simulink model "sub1"  (R2021b)
settings: Solver=FixedStepDiscrete  StartTime=0.0  StopTime=10.0  RelTol=1e-3
libraries: SimulinkLibrary x3
settings Model: Creator=AnusreeSaji  LastModifiedBy=AnusreeSaji

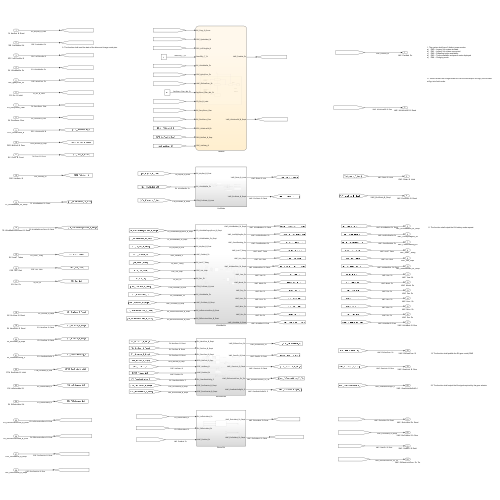
[thumbnail: Simulink's stored preview of the top-level diagram]
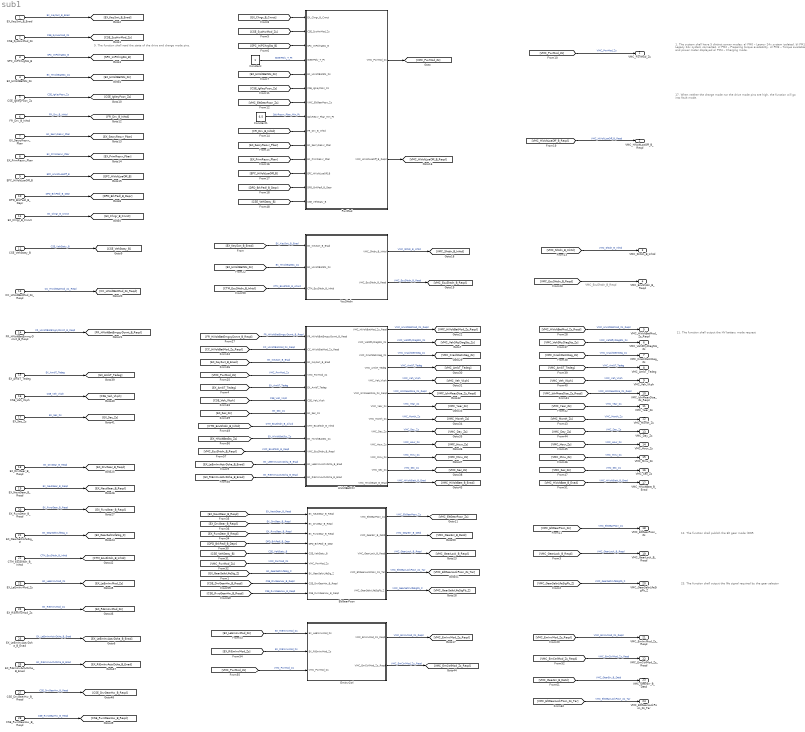
== system sub1 ==
  note: VMC_EcuShtdn_B_Reqd
  note: 11. The function shall output the HV battery mode request
  note: 9. The function shall read the state of the drive and charge mode pins.
  note: 17. When neither the charge mode nor the drive mode pins are high, the function will go into fault mode.
  note: 12. The function shall publish the Elt gear mode (DNR
  note: 1. The system shall have 5 distinct power modes:
      | a)	PM0 – Legacy 24v system isolated.
      | b)	PM1 – Legacy 24v system connected.
      | c)	PM2 – Preparing torque availability.
      | d)	PM3 – Torque available and power meter displayed
      | e)	PM4 – Charging mode.
  note: 23. The function shall output the life signal required by the gear selector
  EX_KeySwt_B_Enad : Inport
  CSE_SysHwMod_Zs : Inport  Port=2
  SPC_IniPChrgSts_B : Inport  Port=3
  EX_HiVoltBatSts_Zs : Inport  Port=4
  CSE_IgKeyPosn_Zs : Inport  Port=5
  FR_Drv_B_Inhtd : Inport  Port=6
  EX_SecryResvr_Pbar : Inport  Port=7
  EX_PrimResvr_Pbar : Inport  Port=8
  EPC_HiVoltLoaOff_B : Inport  Port=9
  DPD_BrkPedl_B_Depr : Inport  Port=10
  EX_Chrgr_B_Cnnct : Inport  Port=11
  CSE_VehStaty_B : Inport  Port=12
  CC_HiVoltBatMod_Zs_Reqd : Inport  Port=13
  FR_HiVoltBatEmgcyDcnnt_B_Reqd : Inport  Port=14
  EX_AmbT_Tedeg : Inport  Port=15
  CSE_Veh_Vkph : Inport  Port=16
  EX_Sec_Zs : Inport  Port=17
  EX_DrvGear_B_Reqd : Inport  Port=18
  EX_NeutGear_B_Reqd : Inport  Port=19
  EX_RvrsGear_B_Reqd : Inport  Port=20
  EX_GearSeltrLifeSig_Z : Inport  Port=21
  CTM_EcuShtdn_B_Inhtd : Inport  Port=22
  EX_LeEmInvMod_Zs : Inport  Port=23
  EX_RiEmInvMod_Zs : Inport  Port=24
  EX_LeEmInvActvDcha_B_Enad : Inport  Port=25
  EX_RiEmInvActvDcha_B_Enad : Inport  Port=26
  CSE_DrvGearHw_B_Reqd : Inport  Port=27
  CSE_RvrsGearHw_B_Reqd : Inport  Port=28
  Constant : Constant
  Constant1 : Constant  Value=6.5
  EltGearPosn : Subsystem
  EmInvCtrl : Subsystem
  HiVoltBatCtrl : Subsystem
  PwrMod : Stateflow chart  TreatAsAtomicUnit=on
  VcuShtdn : Subsystem
  VMC_PwrMod_Zs : Outport  OutDataTypeStr=single
  VMC_HiVoltLoaOff_B_Reqd : Outport  Port=2
  VMC_Shtdn_B_Inhtd : Outport  Port=3
  VMC_EcuShtdn_B_Reqd : Outport  Port=4
  VMC_HiVoltBatMod_Zs_Reqd : Outport  Port=5
  VMC_VehSftyDiagSts_Zs : Outport  Port=6
  VMC_CrashDetnNeg_Zs : Outport  Port=7
  VMC_AmbT_Tedeg : Outport  Port=8
  VMC_Veh_Vkph : Outport  Port=9
  VMC_IslnMeasDisa_Zs_Reqd : Outport  Port=10
  VMC_Year_Zs : Outport  Port=11
  VMC_Month_Zs : Outport  Port=12
  VMC_Day_Zs : Outport  Port=13
  VMC_Hour_Zs : Outport  Port=14
  VMC_Minu_Zs : Outport  Port=15
  VMC_Sec_Zs : Outport  Port=16
  VMC_HiVoltBatt_B_Enad : Outport  Port=17
  VMC_EltGearPosn_Zs : Outport  Port=18
  VMC_GearLock_B_Reqd : Outport  Port=19
  VMC_GearSeltrLifeSigFb_Z : Outport  Port=20
  VMC_EmInvMod_Zs_Reqd : Outport  Port=21
  VMC_EmCtrlMod_Zs_Reqd : Outport  Port=22
  VMC_GearErr_B_Detd : Outport  Port=23
  VMC_EltGearLockPosn_Zs_Tar : Outport  Port=24
  wires:
  CSE_IgKeyPosn_Zs/1 -> [CSE_IgKeyPosn_Zs]  "CSE_IgKeyPosn_Zs"
  SPC_IniPChrgSts_B/1 -> [SPC_IniPChrgSts_B]  "SPC_IniPChrgSts_B"
  [CSE_SysHwMod_Zs] -> PwrMod/2(CSE_SysHwMod_Zs)
  EX_HiVoltBatSts_Zs/1 -> [EX_HiVoltBatSts_Zs]  "EX_HiVoltBatSts_Zs"
  [VMC_PwrMod_Zs] -> EltGearPosn/6(VMC_PwrMod_Zs)  "VMC_PwrMod_Zs"
  [VMC_EltGearPosn_Zs] -> PwrMod/7(VMC_EltGearPosn_Zs)
  CSE_SysHwMod_Zs/1 -> [CSE_SysHwMod_Zs]  "CSE_SysHwMod_Zs"
  PwrMod/1(VMC_PwrMod_Zs) -> [VMC_PwrMod_Zs]
  EX_RvrsGear_B_Reqd/1 -> [EX_RvrsGear_B_Reqd]  "EX_RvrsGear_B_Reqd"
  CSE_RvrsGearHw_B_Reqd/1 -> [CSE_RvrsGearHw_B_Reqd]  "CSE_RvrsGearHw_B_Reqd"
  [CSE_VehStaty_B] -> EltGearPosn/5(CSE_VehStaty_B)  "CSE_VehStaty_B"
  [SPC_IniPChrgSts_B] -> PwrMod/3(SPC_IniPChrgSts_B)
  Constant/1 -> PwrMod/4(SteerPDly_T_Pt)  "SteerPDly_T_Pt"
  [EX_HiVoltBatSts_Zs] -> VcuShtdn/2(EX_HiVoltBatSts_Zs)  "EX_HiVoltBatSts_Zs"
  Constant1/1 -> PwrMod/8(SplyResvr_Pbar_Min_Pt)  "SplyResvr_Pbar_Min_Pt"
  [EX_Chrgr_B_Cnnct] -> PwrMod/1(EX_Chrgr_B_Cnnct)
  HiVoltBatCtrl/12(VMC_Sec_Zs) -> [VMC_Sec_Zs]  "VMC_Sec_Zs"
  VcuShtdn/1(VMC_Shtdn_B_Inhtd) -> [VMC_Shtdn_B_Inhtd]  "VMC_Shtdn_B_Inhtd"
  [CSE_IgKeyPosn_Zs] -> PwrMod/6(CSE_IgKeyPosn_Zs)
  EltGearPosn/5(VMC_GearSeltrLifeSigFb_Z) -> [VMC_GearSeltrLifeSigFb_Z]  "VMC_GearSeltrLifeSigFb_Z"
  CC_HiVoltBatMod_Zs_Reqd/1 -> [CC_HiVoltBatMod_Zs_Reqd]  "CC_HiVoltBatMod_Zs_Reqd"
  [EX_SecryResvr_Pbar] -> PwrMod/10(EX_SecryResvr_Pbar)
  [CSE_Veh_Vkph] -> HiVoltBatCtrl/6(CSE_Veh_Vkph)  "CSE_Veh_Vkph"
  [VMC_PwrMod_Zs] -> EmInvCtrl/3(VMC_PwrMod_Zs)  "VMC_PwrMod_Zs"
  [VMC_PwrMod_Zs] -> VMC_PwrMod_Zs/1  "VMC_PwrMod_Zs"
  [EX_HiVoltBatSts_Zs] -> PwrMod/5(EX_HiVoltBatSts_Zs)
  [DPD_BrkPedl_B_Depr] -> PwrMod/13(DPD_BrkPedl_B_Depr)
  [EX_HiVoltBatSts_Zs] -> HiVoltBatCtrl/9(EX_HiVoltBatSts_Zs)  "EX_HiVoltBatSts_Zs"
  [VMC_Sec_Zs] -> VMC_Sec_Zs/1  "VMC_Sec_Zs"
  EltGearPosn/3(VMC_GearLock_B_Reqd) -> [VMC_GearLock_B_Reqd]  "VMC_GearLock_B_Reqd"
  DPD_BrkPedl_B_Depr/1 -> [DPD_BrkPedl_B_Depr]  "DPD_BrkPedl_B_Depr"
  CSE_VehStaty_B/1 -> [CSE_VehStaty_B]  "CSE_VehStaty_B"
  FR_Drv_B_Inhtd/1 -> [FR_Drv_B_Inhtd]  "FR_Drv_B_Inhtd"
  EX_RiEmInvActvDcha_B_Enad/1 -> [EX_RiEmInvActvDcha_B_Enad]  "EX_RiEmInvActvDcha_B_Enad"
  [VMC_GearLock_B_Reqd] -> VMC_GearLock_B_Reqd/1  "VMC_GearLock_B_Reqd"
  [VMC_EmInvMod_Zs_Reqd] -> VMC_EmInvMod_Zs_Reqd/1  "VMC_EmInvMod_Zs_Reqd"
  [VMC_EltGearLockPosn_Zs_Tar] -> VMC_EltGearLockPosn_Zs_Tar/1  "VMC_EltGearLockPosn_Zs_Tar"
  [VMC_HiVoltLoaOff_B_Reqd] -> VMC_HiVoltLoaOff_B_Reqd/1  "VMC_HiVoltLoaOff_B_Reqd"
  [EX_AmbT_Tedeg] -> HiVoltBatCtrl/5(EX_AmbT_Tedeg)  "EX_AmbT_Tedeg"
  EmInvCtrl/1(VMC_EmInvMod_Zs_Reqd) -> [VMC_EmInvMod_Zs_Reqd]  "VMC_EmInvMod_Zs_Reqd"
  EX_AmbT_Tedeg/1 -> [EX_AmbT_Tedeg]  "EX_AmbT_Tedeg"
  CSE_Veh_Vkph/1 -> [CSE_Veh_Vkph]  "CSE_Veh_Vkph"
  HiVoltBatCtrl/13(VMC_HiVoltBatt_B_Enad) -> [VMC_HiVoltBatt_B_Enad]  "VMC_HiVoltBatt_B_Enad"
  EPC_HiVoltLoaOff_B/1 -> [EPC_HiVoltLoaOff_B]  "EPC_HiVoltLoaOff_B"
  EX_RiEmInvMod_Zs/1 -> [EX_RiEmInvMod_Zs]  "EX_RiEmInvMod_Zs"
  [VMC_EmCtrlMod_Zs_Reqd] -> VMC_EmCtrlMod_Zs_Reqd/1  "VMC_EmCtrlMod_Zs_Reqd"
  CTM_EcuShtdn_B_Inhtd/1 -> [CTM_EcuShtdn_B_Inhtd]  "CTM_EcuShtdn_B_Inhtd"
  [CTM_EcuShtdn_B_Inhtd] -> VcuShtdn/3(CTM_EcuShtdn_B_Inhtd)  "CTM_EcuShtdn_B_Allwd"
  HiVoltBatCtrl/6(VMC_IslnMeasDisa_Zs_Reqd) -> [VMC_IslnMeasDisa_Zs_Reqd]  "VMC_IslnMeasDisa_Zs_Reqd"
  EX_LeEmInvActvDcha_B_Enad/1 -> [EX_LeEmInvActvDcha_B_Enad]  "EX_LeEmInvActvDcha_B_Enad"
  [EX_RiEmInvMod_Zs] -> EmInvCtrl/2(EX_RiEmInvMod_Zs)  "EX_RiEmInvMod_Zs"
  [EX_LeEmInvActvDcha_B_Enad] -> HiVoltBatCtrl/11(EX_LeEmInvActvDcha_B_Enad)  "EX_LeEmInvActvDcha_B_Enad"
  HiVoltBatCtrl/1(VMC_HiVoltBatMod_Zs_Reqd) -> [VMC_HiVoltBatMod_Zs_Reqd]  "VMC_HiVoltBatMod_Zs_Reqd"
  [VMC_CrashDetnNeg_Zs] -> VMC_CrashDetnNeg_Zs/1  "VMC_CrashDetnNeg_Zs"
  [FR_HiVoltBatEmgcyDcnnt_B_Reqd] -> HiVoltBatCtrl/1(FR_HiVoltBatEmgcyDcnnt_B_Reqd)  "FR_HiVoltBatEmgcyDcnnt_B_Reqd"
  [VMC_PwrMod_Zs] -> HiVoltBatCtrl/4(VMC_PwrMod_Zs)  "VMC_PwrMod_Zs"
  [VMC_HiVoltBatMod_Zs_Reqd] -> VMC_HiVoltBatMod_Zs_Reqd/1  "VMC_HiVoltBatMod_Zs_Reqd"
  [EX_LeEmInvMod_Zs] -> EmInvCtrl/1(EX_LeEmInvMod_Zs)  "EX_RiEmInvMod_Zs"
  [VMC_Minu_Zs] -> VMC_Minu_Zs/1  "VMC_Minu_Zs"
  EX_Chrgr_B_Cnnct/1 -> [EX_Chrgr_B_Cnnct]  "EX_Chrgr_B_Cnnct"
  [EX_DrvGear_B_Reqd] -> EltGearPosn/2(EX_DrvGear_B_Reqd)  "EX_DrvGear_B_Reqd"
  [CSE_DrvGearHw_B_Reqd] -> EltGearPosn/8(CSE_DrvGearHw_B_Reqd)  "CSE_DrvGearHw_B_Reqd"
  [EX_RvrsGear_B_Reqd] -> EltGearPosn/3(EX_RvrsGear_B_Reqd)  "EX_RvrsGear_B_Reqd"
  EltGearPosn/1(VMC_EltGearPosn_Zs) -> [VMC_EltGearPosn_Zs]  "VMC_EltGearPosn_Zs"
  FR_HiVoltBatEmgcyDcnnt_B_Reqd/1 -> [FR_HiVoltBatEmgcyDcnnt_B_Reqd]  "FR_HiVoltBatEmgcyDcnnt_B_Reqd"
  CSE_DrvGearHw_B_Reqd/1 -> [CSE_DrvGearHw_B_Reqd]  "CSE_DrvGearHw_B_Reqd"
  [EX_Sec_Zs] -> HiVoltBatCtrl/7(EX_Sec_Zs)  "EX_Sec_Zs"
  HiVoltBatCtrl/5(VMC_Veh_Vkph) -> [VMC_Veh_Vkph]  "VMC_Veh_Vkph"
  EX_KeySwt_B_Enad/1 -> [EX_KeySwt_B_Enad]  "EX_KeySwt_B_Enad"
  HiVoltBatCtrl/2(VMC_VehSftyDiagSts_Zs) -> [VMC_VehSftyDiagSts_Zs]  "VMC_VehSftyDiagSts_Zs"
  EX_LeEmInvMod_Zs/1 -> [EX_LeEmInvMod_Zs]  "EX_LeEmInvMod_Zs"
  [EX_KeySwt_B_Enad] -> HiVoltBatCtrl/3(EX_KeySwt_B_Enad)  "EX_KeySwt_B_Enad"
  HiVoltBatCtrl/3(VMC_CrashDetnNeg_Zs) -> [VMC_CrashDetnNeg_Zs]  "VMC_CrashDetnNeg_Zs"
  HiVoltBatCtrl/4(VMC_AmbT_Tedeg) -> [VMC_AmbT_Tedeg]  "VMC_AmbT_Tedeg"
  EltGearPosn/4(VMC_EltGearLockPosn_Zs_Tar) -> [VMC_EltGearLockPosn_Zs_Tar]  "VMC_EltGearLockPosn_Zs_Tar"
  [VMC_GearErr_B_Detd] -> VMC_GearErr_B_Detd/1  "VMC_GearErr_B_Detd"
  EltGearPosn/2(VMC_GearErr_B_Detd) -> [VMC_GearErr_B_Detd]  "VMC_GearErr_B_Detd"
  [VMC_Veh_Vkph] -> VMC_Veh_Vkph/1  "VMC_Veh_Vkph"
  HiVoltBatCtrl/7(VMC_Year_Zs) -> [VMC_Year_Zs]  "VMC_Year_Zs"
  EX_NeutGear_B_Reqd/1 -> [EX_NeutGear_B_Reqd]  "EX_NeutGear_B_Reqd"
  HiVoltBatCtrl/11(VMC_Minu_Zs) -> [VMC_Minu_Zs]  "VMC_Minu_Zs"
  [VMC_Month_Zs] -> VMC_Month_Zs/1  "VMC_Month_Zs"
  [VMC_AmbT_Tedeg] -> VMC_AmbT_Tedeg/1  "VMC_AmbT_Tedeg"
  EmInvCtrl/2(VMC_EmCtrlMod_Zs_Reqd) -> [VMC_EmCtrlMod_Zs_Reqd]  "VMC_EmCtrlMod_Zs_Reqd"
  [VMC_Day_Zs] -> VMC_Day_Zs/1  "VMC_Day_Zs"
  [CC_HiVoltBatMod_Zs_Reqd] -> HiVoltBatCtrl/2(CC_HiVoltBatMod_Zs_Reqd)  "CC_HiVoltBatMod_Zs_Reqd"
  [VMC_Hour_Zs] -> VMC_Hour_Zs/1  "VMC_Hour_Zs"
  [VMC_Year_Zs] -> VMC_Year_Zs/1  "VMC_Year_Zs"
  [DPD_BrkPedl_B_Depr] -> EltGearPosn/4(DPD_BrkPedl_B_Depr)  "DPD_BrkPedl_B_Depr"
  [VMC_Shtdn_B_Inhtd] -> VMC_Shtdn_B_Inhtd/1  "VMC_Shtdn_B_Inhtd"
  [VMC_HiVoltBatt_B_Enad] -> VMC_HiVoltBatt_B_Enad/1  "VMC_HiVoltBatt_B_Enad"
  [EX_NeutGear_B_Reqd] -> EltGearPosn/1(EX_NeutGear_B_Reqd)  "EX_NeutGear_B_Reqd"
  HiVoltBatCtrl/9(VMC_Day_Zs) -> [VMC_Day_Zs]  "VMC_Day_Zs"
  [CTM_EcuShtdn_B_Inhtd] -> HiVoltBatCtrl/8(CTM_EcuShtdn_B_Inhtd)  "CTM_EcuShtdn_B_Allwd"
  EX_GearSeltrLifeSig_Z/1 -> [EX_GearSeltrLifeSig_Z]  "EX_GearSeltrLifeSig_Z"
  [VMC_EltGearPosn_Zs] -> VMC_EltGearPosn_Zs/1  "VMC_EltGearPosn_Zs"
  HiVoltBatCtrl/8(VMC_Month_Zs) -> [VMC_Month_Zs]  "VMC_Month_Zs"
  EX_DrvGear_B_Reqd/1 -> [EX_DrvGear_B_Reqd]  "EX_DrvGear_B_Reqd"
  PwrMod/2(VMC_HiVoltLoaOff_B_Reqd) -> [VMC_HiVoltLoaOff_B_Reqd]
  VcuShtdn/2(VMC_EcuShtdn_B_Reqd) -> [VMC_EcuShtdn_B_Reqd]  "VMC_EcuShtdn_B_Reqd"
  [CSE_VehStaty_B] -> PwrMod/14(CSE_VehStaty_B)
  [FR_Drv_B_Inhtd] -> PwrMod/9(FR_Drv_B_Inhtd)
  [VMC_IslnMeasDisa_Zs_Reqd] -> VMC_IslnMeasDisa_Zs_Reqd/1  "VMC_IslnMeasDisa_Zs_Reqd"
  [EX_PrimResvr_Pbar] -> PwrMod/11(EX_PrimResvr_Pbar)
  EX_PrimResvr_Pbar/1 -> [EX_PrimResvr_Pbar]  "EX_PrimResvr_Pbar"
  EX_SecryResvr_Pbar/1 -> [EX_SecryResvr_Pbar]  "EX_SecryResvr_Pbar"
  [EX_RiEmInvActvDcha_B_Enad] -> HiVoltBatCtrl/12(EX_RiEmInvActvDcha_B_Enad)  "EX_RiEmInvActvDcha_B_Enad"
  EX_Sec_Zs/1 -> [EX_Sec_Zs]  "EX_Sec_Zs"
  [CSE_RvrsGearHw_B_Reqd] -> EltGearPosn/9(CSE_RvrsGearHw_B_Reqd)  "CSE_RvrsGearHw_B_Reqd"
  [EX_KeySwt_B_Enad] -> VcuShtdn/1(EX_KeySwt_B_Enad)  "EX_KeySwt_B_Enad"
  [EX_GearSeltrLifeSig_Z] -> EltGearPosn/7(EX_GearSeltrLifeSig_Z)  "EX_GearSeltrLifeSig_Z"
  [VMC_EcuShtdn_B_Reqd] -> VMC_EcuShtdn_B_Reqd/1
  HiVoltBatCtrl/10(VMC_Hour_Zs) -> [VMC_Hour_Zs]  "VMC_Hour_Zs"
  [EPC_HiVoltLoaOff_B] -> PwrMod/12(EPC_HiVoltLoaOff_B)
  [VMC_EcuShtdn_B_Reqd] -> HiVoltBatCtrl/10(VMC_EcuShtdn_B_Reqd)  "VMC_EcuShtdn_B_Reqd"
  [VMC_VehSftyDiagSts_Zs] -> VMC_VehSftyDiagSts_Zs/1  "VMC_VehSftyDiagSts_Zs"
  [VMC_GearSeltrLifeSigFb_Z] -> VMC_GearSeltrLifeSigFb_Z/1  "VMC_GearSeltrLifeSigFb_Z"

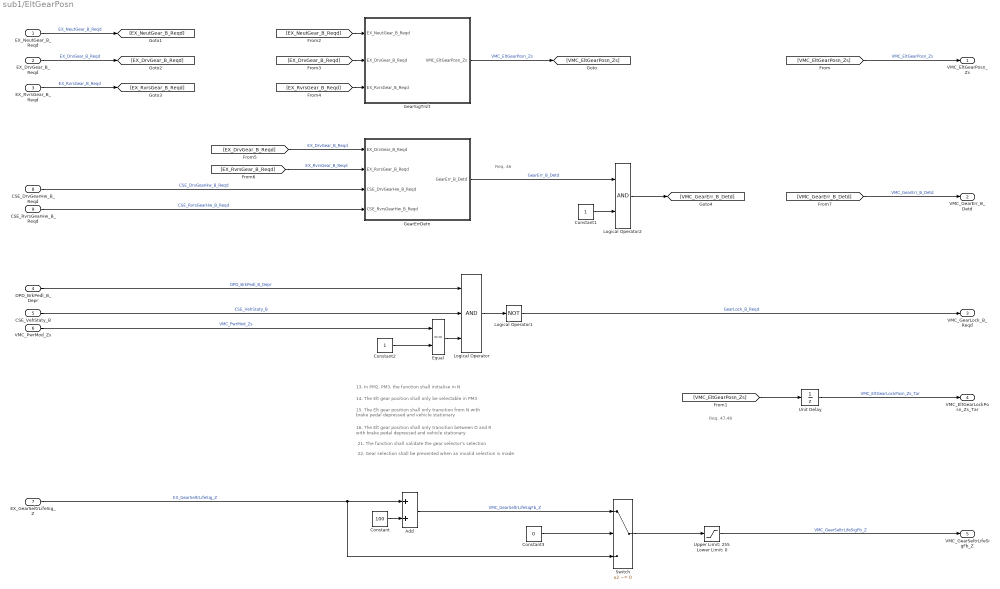
== system sub1/EltGearPosn ==
  note: 13. In PM2, PM3, the function shall initialise in N
  note: 14. The Elt gear position shall only be selectable in PM3
  note: 15. The Elt gear position shall only transition from N with brake pedal depressed and vehicle stationary
  note: 16. The Elt gear position shall only transition between D and R with brake pedal depressed and vehicle stationary
  note: 21. The function shall validate the gear selector’s selection
  note: 22. Gear selection shall be prevented when an invalid selection is made
  note: Req. 46
  note: Req. 47,48
  EX_NeutGear_B_Reqd : Inport
  EX_DrvGear_B_Reqd : Inport  Port=2
  EX_RvrsGear_B_Reqd : Inport  Port=3
  DPD_BrkPedl_B_Depr : Inport  Port=4
  CSE_VehStaty_B : Inport  Port=5
  VMC_PwrMod_Zs : Inport  Port=6
  EX_GearSeltrLifeSig_Z : Inport  Port=7
  CSE_DrvGearHw_B_Reqd : Inport  Port=8
  CSE_RvrsGearHw_B_Reqd : Inport  Port=9
  Add : Sum
  Constant : Constant  Value=100
  Constant1 : Constant
  Constant2 : Constant
  Constant3 : Constant  Value=0
  Equal : RelationalOperator  Operator===  OutDataTypeStr=boolean  RndMeth=Simplest
  GearErrDetn : Subsystem
  GearSigTrslt : Subsystem
  Logical Operator : Logic  Inputs=3  AllPortsSameDT=off  OutDataTypeStr=boolean
  Logical Operator1 : Logic  Operator=NOT  AllPortsSameDT=off  OutDataTypeStr=boolean
  Logical Operator2 : Logic  AllPortsSameDT=off  OutDataTypeStr=boolean
  Switch : Switch  Criteria=u2 ~= 0
  Unit Delay : UnitDelay  SampleTime=-1  HasFrameUpgradeWarning=on
  Upper Limit: 255 Lower Limit: 0 : Saturate  UpperLimit=100  LowerLimit=0
  VMC_EltGearPosn_Zs : Outport
  VMC_GearErr_B_Detd : Outport  Port=2
  VMC_GearLock_B_Reqd : Outport  Port=3
  VMC_EltGearLockPosn_Zs_Tar : Outport  Port=4
  VMC_GearSeltrLifeSigFb_Z : Outport  Port=5
  wires:
  Constant3/1 -> Switch/2
  Switch/1 -> Upper Limit: 255 Lower Limit: 0/1
  Add/1 -> Switch/1  "VMC_GearSeltrLifeSigFb_Z"
  Logical Operator2/1 -> [VMC_GearErr_B_Detd]
  [VMC_GearErr_B_Detd] -> VMC_GearErr_B_Detd/1  "VMC_GearErr_B_Detd"
  Constant1/1 -> Logical Operator2/2
  GearErrDetn/1(GearErr_B_Detd) -> Logical Operator2/1  "GearErr_B_Detd"
  CSE_DrvGearHw_B_Reqd/1 -> GearErrDetn/3(CSE_DrvGearHw_B_Reqd)  "CSE_DrvGearHw_B_Reqd"
  CSE_RvrsGearHw_B_Reqd/1 -> GearErrDetn/4(CSE_RvrsGearHw_B_Reqd)  "CSE_RvrsGearHw_B_Reqd"
  [EX_RvrsGear_B_Reqd] -> GearErrDetn/2(EX_RvrsGear_B_Reqd)  "EX_RvrsGear_B_Reqd"
  [EX_DrvGear_B_Reqd] -> GearErrDetn/1(EX_DrvGear_B_Reqd)  "EX_DrvGear_B_Reqd"
  [EX_RvrsGear_B_Reqd] -> GearSigTrslt/3(EX_RvrsGear_B_Reqd)
  [EX_DrvGear_B_Reqd] -> GearSigTrslt/2(EX_DrvGear_B_Reqd)
  [EX_NeutGear_B_Reqd] -> GearSigTrslt/1(EX_NeutGear_B_Reqd)
  Unit Delay/1 -> VMC_EltGearLockPosn_Zs_Tar/1  "VMC_EltGearLockPosn_Zs_Tar"
  [VMC_EltGearPosn_Zs] -> Unit Delay/1
  [VMC_EltGearPosn_Zs] -> VMC_EltGearPosn_Zs/1  "VMC_EltGearPosn_Zs"
  Upper Limit: 255 Lower Limit: 0/1 -> VMC_GearSeltrLifeSigFb_Z/1  "VMC_GearSeltrLifeSigFb_Z"
  Constant/1 -> Add/2
  EX_GearSeltrLifeSig_Z/1 -> Add/1, Switch/3  "EX_GearSeltrLifeSig_Z"
  EX_RvrsGear_B_Reqd/1 -> [EX_RvrsGear_B_Reqd]  "EX_RvrsGear_B_Reqd"
  EX_DrvGear_B_Reqd/1 -> [EX_DrvGear_B_Reqd]  "EX_DrvGear_B_Reqd"
  Logical Operator1/1 -> VMC_GearLock_B_Reqd/1  "GearLock_B_Reqd"
  VMC_PwrMod_Zs/1 -> Equal/1  "VMC_PwrMod_Zs"
  Logical Operator/1 -> Logical Operator1/1
  CSE_VehStaty_B/1 -> Logical Operator/2  "CSE_VehStaty_B"
  GearSigTrslt/1(VMC_EltGearPosn_Zs) -> [VMC_EltGearPosn_Zs]  "VMC_EltGearPosn_Zs"
  Equal/1 -> Logical Operator/3
  Constant2/1 -> Equal/2
  EX_NeutGear_B_Reqd/1 -> [EX_NeutGear_B_Reqd]  "EX_NeutGear_B_Reqd"
  DPD_BrkPedl_B_Depr/1 -> Logical Operator/1  "DPD_BrkPedl_B_Depr"

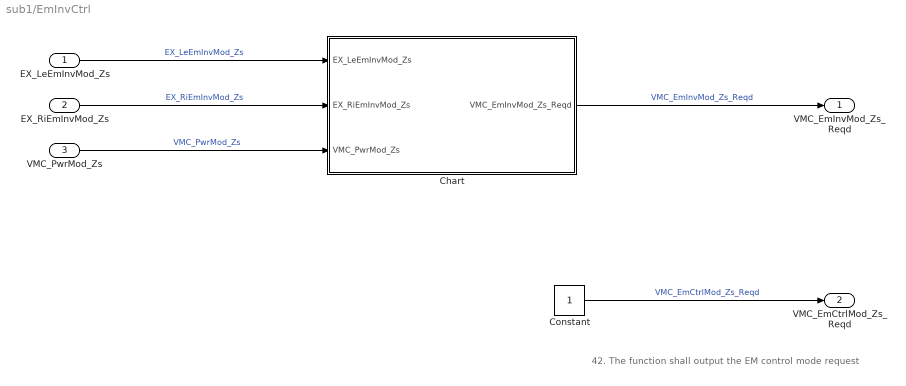
== system sub1/EmInvCtrl ==
  note: 42. The function shall output the EM control mode request
  EX_LeEmInvMod_Zs : Inport
  EX_RiEmInvMod_Zs : Inport  Port=2
  VMC_PwrMod_Zs : Inport  Port=3
  Chart : Stateflow chart  TreatAsAtomicUnit=on
  Constant : Constant
  VMC_EmInvMod_Zs_Reqd : Outport
  VMC_EmCtrlMod_Zs_Reqd : Outport  Port=2
  wires:
  Constant/1 -> VMC_EmCtrlMod_Zs_Reqd/1  "VMC_EmCtrlMod_Zs_Reqd"
  VMC_PwrMod_Zs/1 -> Chart/3(VMC_PwrMod_Zs)  "VMC_PwrMod_Zs"
  EX_LeEmInvMod_Zs/1 -> Chart/1(EX_LeEmInvMod_Zs)  "EX_LeEmInvMod_Zs"
  EX_RiEmInvMod_Zs/1 -> Chart/2(EX_RiEmInvMod_Zs)  "EX_RiEmInvMod_Zs"
  Chart/1(VMC_EmInvMod_Zs_Reqd) -> VMC_EmInvMod_Zs_Reqd/1  "VMC_EmInvMod_Zs_Reqd"

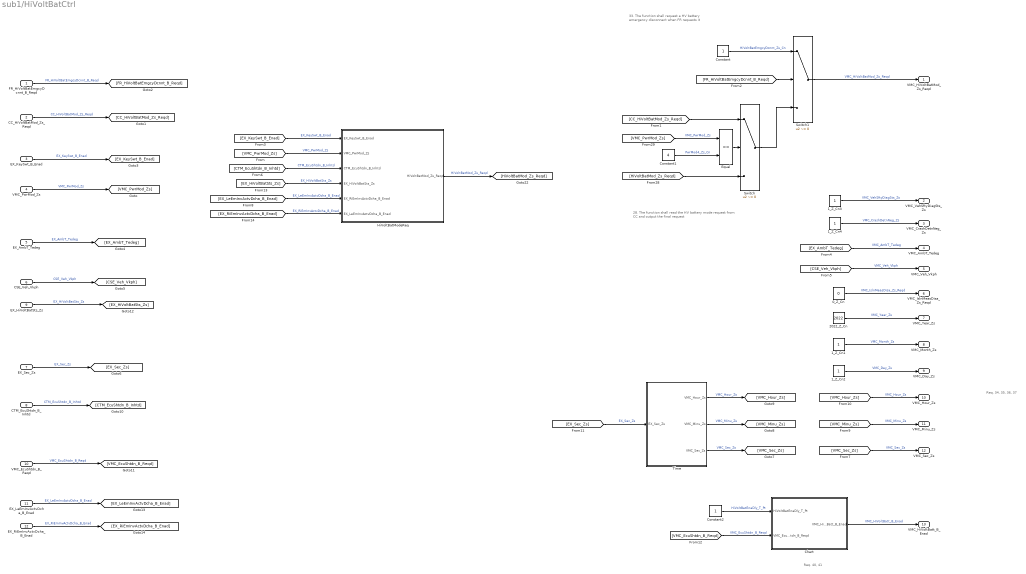
== system sub1/HiVoltBatCtrl ==
  note: 28. The function shall read the HV battery mode request from CC and output the final request
  note: 33. The function shall request a HV battery emergency disconnect when FR requests it
  note: Req. 34, 35, 36, 37
  note: Req. 40, 41
  FR_HiVoltBatEmgcyDcnnt_B_Reqd : Inport
  CC_HiVoltBatMod_Zs_Reqd : Inport  Port=2
  EX_KeySwt_B_Enad : Inport  Port=3
  VMC_PwrMod_Zs : Inport  Port=4
  EX_AmbT_Tedeg : Inport  Port=5
  CSE_Veh_Vkph : Inport  Port=6
  EX_Sec_Zs : Inport  Port=7
  CTM_EcuShtdn_B_Inhtd : Inport  Port=8
  EX_HiVoltBatSts_Zs : Inport  Port=9
  VMC_EcuShtdn_B_Reqd : Inport  Port=10
  EX_LeEmInvActvDcha_B_Enad : Inport  Port=11
  EX_RiEmInvActvDcha_B_Enad : Inport  Port=12
  0_Z_Cn : Constant  Value=0
  1_Z_Cn{1..4} (4 alike) : Constant
  2022_Z_Cn : Constant  Value=2022
  Chart : Stateflow chart  TreatAsAtomicUnit=on
  Constant : Constant
  Constant1 : Constant  Value=4
  Constant2 : Constant
  Equal : RelationalOperator  Operator===  OutDataTypeStr=boolean  RndMeth=Simplest
  HiVoltBatModeReq : Stateflow chart  TreatAsAtomicUnit=on
  Switch : Switch  Criteria=u2 ~= 0
  Switch1 : Switch  Criteria=u2 ~= 0
  Time : Subsystem
  VMC_HiVoltBatMod_Zs_Reqd : Outport
  VMC_VehSftyDiagSts_Zs : Outport  Port=2
  VMC_CrashDetnNeg_Zs : Outport  Port=3
  VMC_AmbT_Tedeg : Outport  Port=4
  VMC_Veh_Vkph : Outport  Port=5
  VMC_IslnMeasDisa_Zs_Reqd : Outport  Port=6
  VMC_Year_Zs : Outport  Port=7
  VMC_Month_Zs : Outport  Port=8
  VMC_Day_Zs : Outport  Port=9
  VMC_Hour_Zs : Outport  Port=10
  VMC_Minu_Zs : Outport  Port=11
  VMC_Sec_Zs : Outport  Port=12
  VMC_HiVoltBatt_B_Enad : Outport  Port=13
  wires:
  [EX_RiEmInvActvDcha_B_Enad] -> HiVoltBatModeReq/6(EX_LeEmInvActvDcha_B_Enad)  "EX_RiEmInvActvDcha_B_Enad"
  [EX_LeEmInvActvDcha_B_Enad] -> HiVoltBatModeReq/5(EX_RiEmInvActvDcha_B_Enad)  "EX_LeEmInvActvDcha_B_Enad"
  EX_RiEmInvActvDcha_B_Enad/1 -> [EX_RiEmInvActvDcha_B_Enad]  "EX_RiEmInvActvDcha_B_Enad"
  EX_LeEmInvActvDcha_B_Enad/1 -> [EX_LeEmInvActvDcha_B_Enad]  "EX_LeEmInvActvDcha_B_Enad"
  VMC_EcuShtdn_B_Reqd/1 -> [VMC_EcuShtdn_B_Reqd]  "VMC_EcuShtdn_B_Reqd"
  [VMC_EcuShtdn_B_Reqd] -> Chart/2(VMC_EcuShtdn_B_Reqd)  "VMC_EcuShtdn_B_Reqd"
  [EX_HiVoltBatSts_Zs] -> HiVoltBatModeReq/4(EX_HiVoltBatSts_Zs)  "EX_HiVoltBatSts_Zs"
  EX_HiVoltBatSts_Zs/1 -> [EX_HiVoltBatSts_Zs]  "EX_HiVoltBatSts_Zs"
  Chart/1(VMC_HiVoltBatt_B_Enad) -> VMC_HiVoltBatt_B_Enad/1  "VMC_HiVoltBatt_B_Enad"
  Constant2/1 -> Chart/1(HiVoltBatEnaDly_T_Pt)  "HiVoltBatEnaDly_T_Pt"
  [CTM_EcuShtdn_B_Inhtd] -> HiVoltBatModeReq/3(CTM_EcuShtdn_B_Inhtd)  "CTM_EcuShtdn_B_Inhtd"
  CTM_EcuShtdn_B_Inhtd/1 -> [CTM_EcuShtdn_B_Inhtd]  "CTM_EcuShtdn_B_Inhtd"
  1_Z_Cn1/1 -> VMC_Month_Zs/1  "VMC_Month_Zs"
  2022_Z_Cn/1 -> VMC_Year_Zs/1  "VMC_Year_Zs"
  1_Z_Cn2/1 -> VMC_Day_Zs/1  "VMC_Day_Zs"
  Time/3(VMC_Sec_Zs) -> [VMC_Sec_Zs]  "VMC_Sec_Zs"
  Time/2(VMC_Minu_Zs) -> [VMC_Minu_Zs]  "VMC_Minu_Zs"
  Time/1(VMC_Hour_Zs) -> [VMC_Hour_Zs]  "VMC_Hour_Zs"
  [EX_Sec_Zs] -> Time/1(EX_Sec_Zs)  "EX_Sec_Zs"
  [VMC_Hour_Zs] -> VMC_Hour_Zs/1  "VMC_Hour_Zs"
  [VMC_Minu_Zs] -> VMC_Minu_Zs/1  "VMC_Minu_Zs"
  [VMC_Sec_Zs] -> VMC_Sec_Zs/1  "VMC_Sec_Zs"
  EX_Sec_Zs/1 -> [EX_Sec_Zs]  "EX_Sec_Zs"
  0_Z_Cn/1 -> VMC_IslnMeasDisa_Zs_Reqd/1  "VMC_IslnMeasDisa_Zs_Reqd"
  [CSE_Veh_Vkph] -> VMC_Veh_Vkph/1  "VMC_Veh_Vkph"
  CSE_Veh_Vkph/1 -> [CSE_Veh_Vkph]  "CSE_Veh_Vkph"
  [EX_AmbT_Tedeg] -> VMC_AmbT_Tedeg/1  "VMC_AmbT_Tedeg"
  EX_AmbT_Tedeg/1 -> [EX_AmbT_Tedeg]  "EX_AmbT_Tedeg"
  1_Z_Cn4/1 -> VMC_CrashDetnNeg_Zs/1  "VMC_CrashDetnNeg_Zs"
  1_Z_Cn3/1 -> VMC_VehSftyDiagSts_Zs/1  "VMC_VehSftyDiagSts_Zs"
  [EX_KeySwt_B_Enad] -> HiVoltBatModeReq/1(EX_KeySwt_B_Enad)  "EX_KeySwt_B_Enad"
  [FR_HiVoltBatEmgcyDcnnt_B_Reqd] -> Switch1/2
  FR_HiVoltBatEmgcyDcnnt_B_Reqd/1 -> [FR_HiVoltBatEmgcyDcnnt_B_Reqd]  "FR_HiVoltBatEmgcyDcnnt_B_Reqd"
  [CC_HiVoltBatMod_Zs_Reqd] -> Switch/1
  CC_HiVoltBatMod_Zs_Reqd/1 -> [CC_HiVoltBatMod_Zs_Reqd]  "CC_HiVoltBatMod_Zs_Reqd"
  EX_KeySwt_B_Enad/1 -> [EX_KeySwt_B_Enad]  "EX_KeySwt_B_Enad"
  [VMC_PwrMod_Zs] -> HiVoltBatModeReq/2(VMC_PwrMod_Zs)  "VMC_PwrMod_Zs"
  VMC_PwrMod_Zs/1 -> [VMC_PwrMod_Zs]  "VMC_PwrMod_Zs"
  Constant1/1 -> Equal/2  "PwrMod4_Zs_Cn"
  HiVoltBatModeReq/1(HiVoltBatMod_Zs_Reqd) -> [HiVoltBatMod_Zs_Reqd]  "HiVoltBatMod_Zs_Reqd"
  Switch/1 -> Switch1/3
  [HiVoltBatMod_Zs_Reqd] -> Switch/3
  Equal/1 -> Switch/2
  [VMC_PwrMod_Zs] -> Equal/1  "VMC_PwrMod_Zs"
  Switch1/1 -> VMC_HiVoltBatMod_Zs_Reqd/1  "VMC_HiVoltBatMod_Zs_Reqd"
  Constant/1 -> Switch1/1  "HiVoltBatEmgcyDcnnt_Zs_Cn"

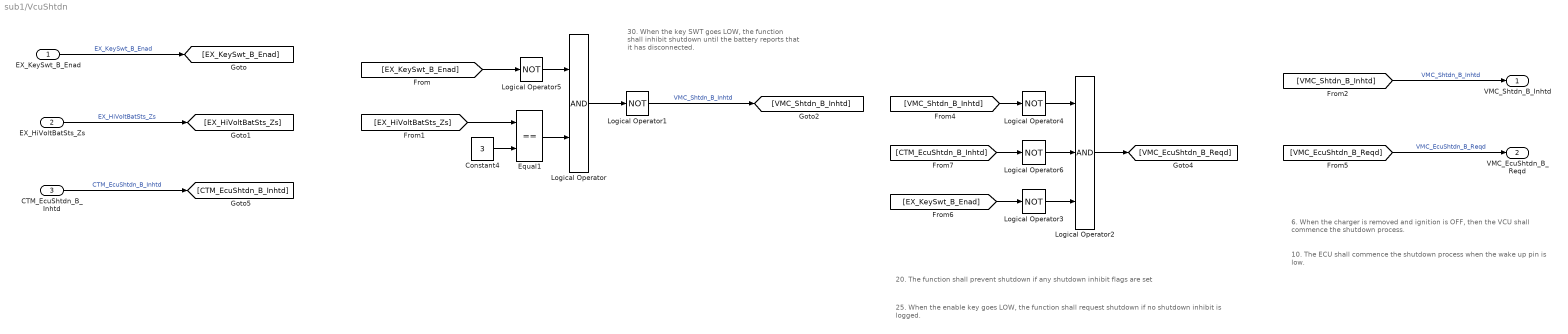
== system sub1/VcuShtdn ==
  note: 10. The ECU shall commence the shutdown process when the wake up pin is low.
  note: 6. When the charger is removed and ignition is OFF, then the VCU shall commence the shutdown process.
  note: 30. When the key SWT goes LOW, the function shall inhibit shutdown until the battery reports that it has disconnected.
  note: 20. The function shall prevent shutdown if any shutdown inhibit flags are set
  note: 25. When the enable key goes LOW, the function shall request shutdown if no shutdown inhibit is logged.
  EX_KeySwt_B_Enad : Inport
  EX_HiVoltBatSts_Zs : Inport  Port=2
  CTM_EcuShtdn_B_Inhtd : Inport  Port=3
  Constant4 : Constant  Value=3
  Equal1 : RelationalOperator  Operator===  OutDataTypeStr=boolean  RndMeth=Simplest
  Logical Operator : Logic  AllPortsSameDT=off  OutDataTypeStr=boolean
  Logical Operator{1,3..6} (5 alike) : Logic  Operator=NOT  AllPortsSameDT=off  OutDataTypeStr=boolean
  Logical Operator2 : Logic  Inputs=3  AllPortsSameDT=off  OutDataTypeStr=boolean
  VMC_Shtdn_B_Inhtd : Outport
  VMC_EcuShtdn_B_Reqd : Outport  Port=2
  wires:
  [CTM_EcuShtdn_B_Inhtd] -> Logical Operator6/1
  CTM_EcuShtdn_B_Inhtd/1 -> [CTM_EcuShtdn_B_Inhtd]  "CTM_EcuShtdn_B_Inhtd"
  Logical Operator3/1 -> Logical Operator2/3
  Logical Operator2/1 -> [VMC_EcuShtdn_B_Reqd]
  Logical Operator4/1 -> Logical Operator2/1
  [VMC_Shtdn_B_Inhtd] -> Logical Operator4/1
  [EX_KeySwt_B_Enad] -> Logical Operator3/1
  [VMC_EcuShtdn_B_Reqd] -> VMC_EcuShtdn_B_Reqd/1  "VMC_EcuShtdn_B_Reqd"
  Logical Operator6/1 -> Logical Operator2/2
  [VMC_Shtdn_B_Inhtd] -> VMC_Shtdn_B_Inhtd/1  "VMC_Shtdn_B_Inhtd"
  [EX_HiVoltBatSts_Zs] -> Equal1/1
  [EX_KeySwt_B_Enad] -> Logical Operator5/1
  Logical Operator/1 -> Logical Operator1/1
  Logical Operator1/1 -> [VMC_Shtdn_B_Inhtd]  "VMC_Shtdn_B_Inhtd"
  EX_KeySwt_B_Enad/1 -> [EX_KeySwt_B_Enad]  "EX_KeySwt_B_Enad"
  Constant4/1 -> Equal1/2
  Equal1/1 -> Logical Operator/2
  Logical Operator5/1 -> Logical Operator/1
  EX_HiVoltBatSts_Zs/1 -> [EX_HiVoltBatSts_Zs]  "EX_HiVoltBatSts_Zs"

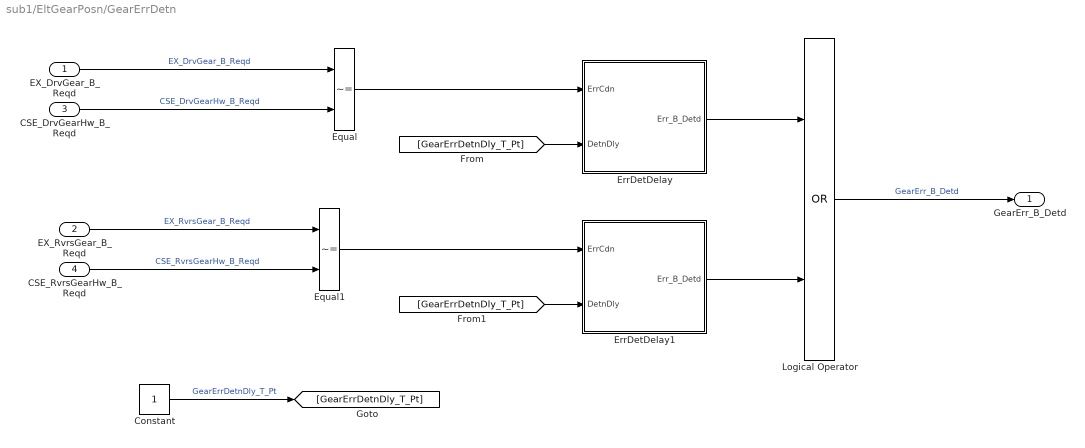
== system sub1/EltGearPosn/GearErrDetn ==
  EX_DrvGear_B_Reqd : Inport
  EX_RvrsGear_B_Reqd : Inport  Port=2
  CSE_DrvGearHw_B_Reqd : Inport  Port=3
  CSE_RvrsGearHw_B_Reqd : Inport  Port=4
  Constant : Constant
  Equal : RelationalOperator  Operator=~=  OutDataTypeStr=boolean  RndMeth=Simplest
  Equal1 : RelationalOperator  Operator=~=  OutDataTypeStr=boolean  RndMeth=Simplest
  ErrDetDelay : Stateflow chart  TreatAsAtomicUnit=on
  ErrDetDelay1 : Stateflow chart  TreatAsAtomicUnit=on
  Logical Operator : Logic  Operator=OR  AllPortsSameDT=off  OutDataTypeStr=boolean
  GearErr_B_Detd : Outport
  wires:
  [GearErrDetnDly_T_Pt] -> ErrDetDelay1/2(DetnDly)
  [GearErrDetnDly_T_Pt] -> ErrDetDelay/2(DetnDly)
  Constant/1 -> [GearErrDetnDly_T_Pt]  "GearErrDetnDly_T_Pt"
  Equal1/1 -> ErrDetDelay1/1(ErrCdn)
  CSE_RvrsGearHw_B_Reqd/1 -> Equal1/2  "CSE_RvrsGearHw_B_Reqd"
  EX_RvrsGear_B_Reqd/1 -> Equal1/1  "EX_RvrsGear_B_Reqd"
  Equal/1 -> ErrDetDelay/1(ErrCdn)
  CSE_DrvGearHw_B_Reqd/1 -> Equal/2  "CSE_DrvGearHw_B_Reqd"
  EX_DrvGear_B_Reqd/1 -> Equal/1  "EX_DrvGear_B_Reqd"
  Logical Operator/1 -> GearErr_B_Detd/1  "GearErr_B_Detd"
  ErrDetDelay1/1(Err_B_Detd) -> Logical Operator/2
  ErrDetDelay/1(Err_B_Detd) -> Logical Operator/1

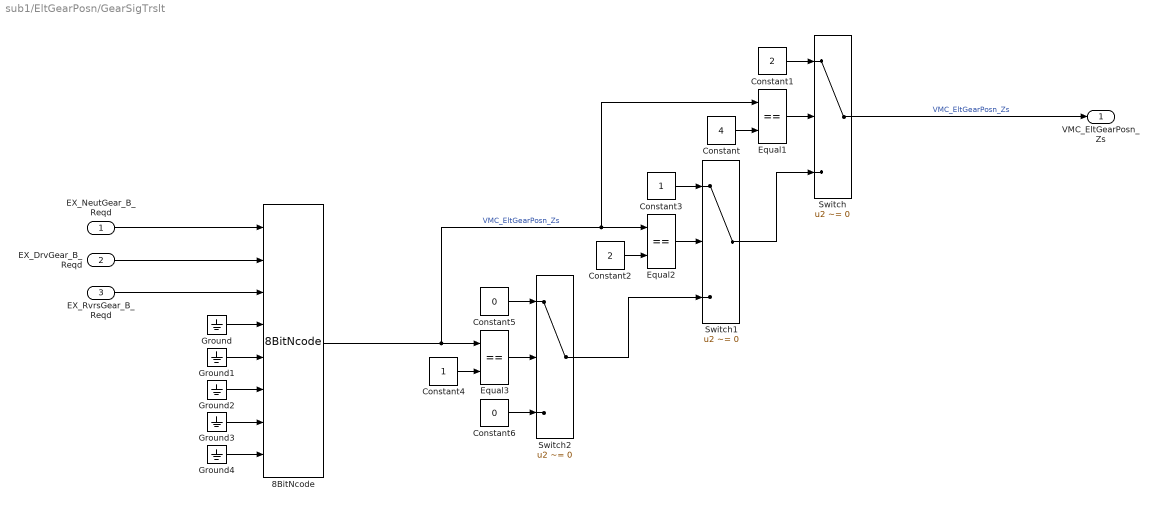
== system sub1/EltGearPosn/GearSigTrslt ==
  EX_NeutGear_B_Reqd : Inport
  EX_DrvGear_B_Reqd : Inport  Port=2
  EX_RvrsGear_B_Reqd : Inport  Port=3
  8BitNcode : SimulinkLibrary/8BitNcode  SystemSampleTime=-1  VariantActivationTime=update diagram  Latency=0  AutoFrameSizeCalculation=off
  Constant : Constant  Value=4
  Constant1 : Constant  Value=2
  Constant2 : Constant  Value=2
  Constant3 : Constant
  Constant4 : Constant
  Constant5 : Constant  Value=0
  Constant6 : Constant  Value=0
  Equal1 : RelationalOperator  Operator===  OutDataTypeStr=boolean  RndMeth=Simplest
  Equal2 : RelationalOperator  Operator===  OutDataTypeStr=boolean  RndMeth=Simplest
  Equal3 : RelationalOperator  Operator===  OutDataTypeStr=boolean  RndMeth=Simplest
  Ground{,1..4} (5 alike) : Ground
  Switch : Switch  Criteria=u2 ~= 0
  Switch1 : Switch  Criteria=u2 ~= 0
  Switch2 : Switch  Criteria=u2 ~= 0
  VMC_EltGearPosn_Zs : Outport
  wires:
  EX_RvrsGear_B_Reqd/1 -> 8BitNcode/3
  EX_NeutGear_B_Reqd/1 -> 8BitNcode/1
  Constant/1 -> Equal1/2
  Ground3/1 -> 8BitNcode/7
  Equal1/1 -> Switch/2
  Switch1/1 -> Switch/3
  Constant1/1 -> Switch/1
  Constant5/1 -> Switch2/1
  Equal3/1 -> Switch2/2
  Ground1/1 -> 8BitNcode/5
  Constant3/1 -> Switch1/1
  Constant4/1 -> Equal3/2
  Equal2/1 -> Switch1/2
  Ground2/1 -> 8BitNcode/6
  Ground/1 -> 8BitNcode/4
  EX_DrvGear_B_Reqd/1 -> 8BitNcode/2
  8BitNcode/1 -> Equal2/1, Equal1/1, Equal3/1  "VMC_EltGearPosn_Zs"
  Switch2/1 -> Switch1/3
  Ground4/1 -> 8BitNcode/8
  Constant2/1 -> Equal2/2
  Constant6/1 -> Switch2/3
  Switch/1 -> VMC_EltGearPosn_Zs/1  "VMC_EltGearPosn_Zs"

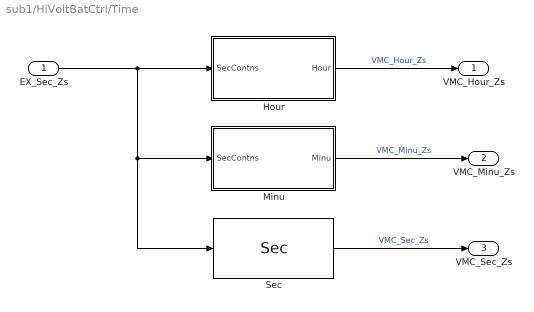
== system sub1/HiVoltBatCtrl/Time ==
  EX_Sec_Zs : Inport
  Hour : Subsystem
  Minu : Subsystem
  "Sec " : SimulinkLibrary/Sec  SystemSampleTime=-1  VariantActivationTime=update diagram  Latency=0  AutoFrameSizeCalculation=off
  VMC_Hour_Zs : Outport
  VMC_Minu_Zs : Outport  Port=2
  VMC_Sec_Zs : Outport  Port=3
  wires:
  "Sec "/1 -> VMC_Sec_Zs/1  "VMC_Sec_Zs"
  Hour/1(Hour) -> VMC_Hour_Zs/1  "VMC_Hour_Zs"
  EX_Sec_Zs/1 -> Hour/1(SecContns), Minu/1(SecContns), "Sec "/1
  Minu/1(Minu) -> VMC_Minu_Zs/1  "VMC_Minu_Zs"

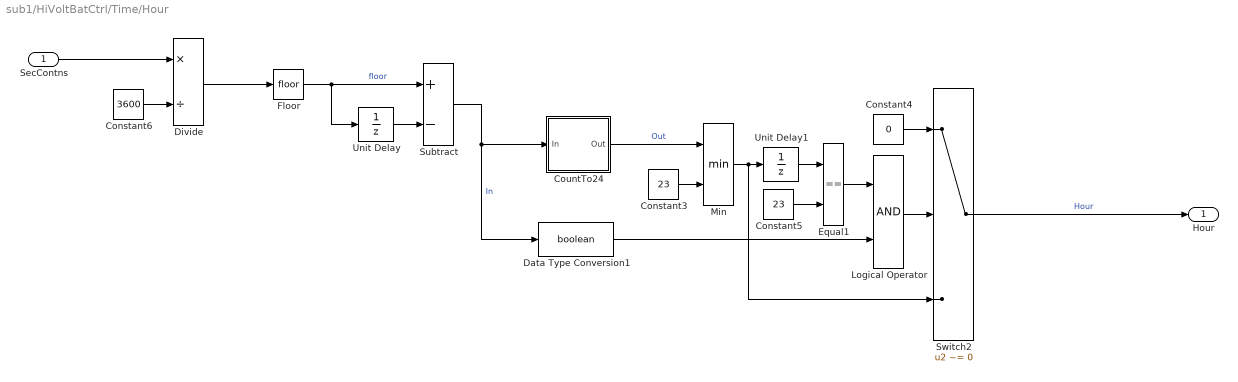
== system sub1/HiVoltBatCtrl/Time/Hour ==
  SecContns : Inport
  Constant3 : Constant  Value=23
  Constant4 : Constant  Value=0
  Constant5 : Constant  Value=23
  Constant6 : Constant  Value=3600
  CountTo24 : Stateflow chart  TreatAsAtomicUnit=on
  Data Type Conversion1 : DataTypeConversion  OutDataTypeStr=boolean
  Divide : Product  Inputs=*/
  Equal1 : RelationalOperator  Operator===  OutDataTypeStr=boolean  RndMeth=Simplest
  Floor : Rounding
  Logical Operator : Logic  AllPortsSameDT=off  OutDataTypeStr=boolean
  Min : MinMax  Inputs=2
  Subtract : Sum  Inputs=+-
  Switch2 : Switch  Criteria=u2 ~= 0
  Unit Delay : UnitDelay  SampleTime=-1  HasFrameUpgradeWarning=on
  Unit Delay1 : UnitDelay  SampleTime=-1  HasFrameUpgradeWarning=on
  Hour : Outport
  wires:
  Data Type Conversion1/1 -> Logical Operator/2
  Constant3/1 -> Min/2
  Min/1 -> Switch2/3, Unit Delay1/1
  Logical Operator/1 -> Switch2/2
  CountTo24/1(Out) -> Min/1  "Out"
  Constant4/1 -> Switch2/1
  SecContns/1 -> Divide/1
  Constant5/1 -> Equal1/2
  Subtract/1 -> Data Type Conversion1/1, CountTo24/1(In)  "In"
  Unit Delay/1 -> Subtract/2
  Unit Delay1/1 -> Equal1/1
  Divide/1 -> Floor/1
  Switch2/1 -> Hour/1  "Hour"
  Equal1/1 -> Logical Operator/1
  Floor/1 -> Subtract/1, Unit Delay/1  "floor"
  Constant6/1 -> Divide/2

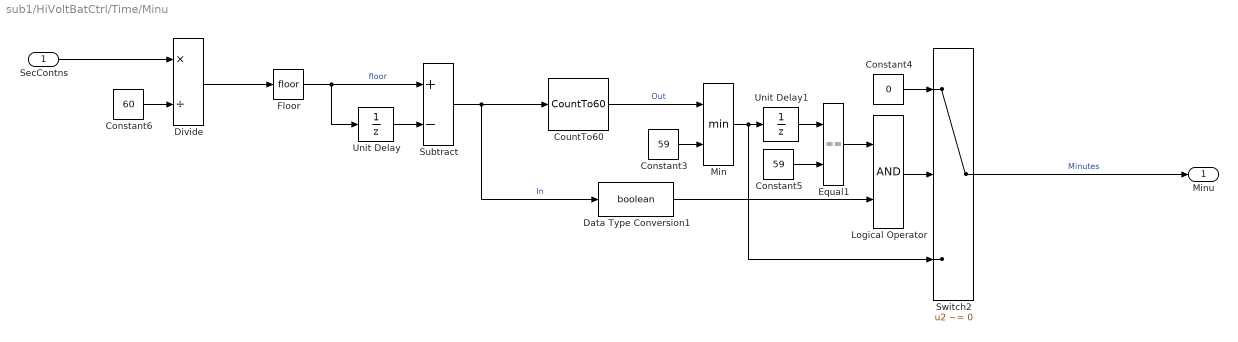
== system sub1/HiVoltBatCtrl/Time/Minu ==
  SecContns : Inport
  Constant3 : Constant  Value=59
  Constant4 : Constant  Value=0
  Constant5 : Constant  Value=59
  Constant6 : Constant  Value=60
  CountTo60 : SimulinkLibrary/Sec/CountTo60  SystemSampleTime=-1  VariantActivationTime=update diagram  Latency=0  AutoFrameSizeCalculation=off
  Data Type Conversion1 : DataTypeConversion  OutDataTypeStr=boolean
  Divide : Product  Inputs=*/
  Equal1 : RelationalOperator  Operator===  OutDataTypeStr=boolean  RndMeth=Simplest
  Floor : Rounding
  Logical Operator : Logic  AllPortsSameDT=off  OutDataTypeStr=boolean
  Min : MinMax  Inputs=2
  Subtract : Sum  Inputs=+-
  Switch2 : Switch  Criteria=u2 ~= 0
  Unit Delay : UnitDelay  SampleTime=-1  HasFrameUpgradeWarning=on
  Unit Delay1 : UnitDelay  SampleTime=-1  HasFrameUpgradeWarning=on
  Minu : Outport
  wires:
  Data Type Conversion1/1 -> Logical Operator/2
  Constant6/1 -> Divide/2
  Floor/1 -> Unit Delay/1, Subtract/1  "floor"
  Equal1/1 -> Logical Operator/1
  Switch2/1 -> Minu/1  "Minutes"
  Divide/1 -> Floor/1
  Unit Delay1/1 -> Equal1/1
  Unit Delay/1 -> Subtract/2
  Subtract/1 -> CountTo60/1, Data Type Conversion1/1  "In"
  Constant5/1 -> Equal1/2
  SecContns/1 -> Divide/1
  Constant4/1 -> Switch2/1
  CountTo60/1 -> Min/1  "Out"
  Logical Operator/1 -> Switch2/2
  Min/1 -> Unit Delay1/1, Switch2/3
  Constant3/1 -> Min/2

== stateflow chart sub1/EltGearPosn/GearErrDetn/ErrDetDelay ==
  state No_error
    entry:
    Err_B_Detd = 0;
  state Error_Det_Review
    entry:
    Err_B_Detd = 0;
  state Error_Confirmed
    entry:
    Err_B_Detd = 1;
  (default) -> No_error
  (junction 11) -> No_error
  (junction 9) -> (junction 11) : [ErrCdn == 0]
  No_error -> Error_Det_Review : [ErrCdn == 1] % Error condition is true
  Error_Det_Review -> (junction 9) [order 1]
  (junction 25) -> (junction 9)
  Error_Det_Review -> (junction 20) [order 2] : [after (DetnDly, sec)] % Detction delay
  (junction 20) -> Error_Confirmed : [ErrCdn == 1 ]
  Error_Confirmed -> (junction 25)
  data: Err_B_Detd output; ErrCdn input; DetnDly input

== stateflow chart sub1/EltGearPosn/GearErrDetn/ErrDetDelay1 ==
  state No_error
    entry:
    Err_B_Detd = 0;
  state Error_Det_Review
    entry:
    Err_B_Detd = 0;
  state Error_Confirmed
    entry:
    Err_B_Detd = 1;
  (default) -> No_error
  (junction 11) -> No_error
  (junction 9) -> (junction 11) : [ErrCdn == 0]
  No_error -> Error_Det_Review : [ErrCdn == 1] % Error condition is true
  Error_Det_Review -> (junction 9) [order 1]
  (junction 25) -> (junction 9)
  Error_Det_Review -> (junction 20) [order 2] : [after (DetnDly, sec)] % Detction delay
  (junction 20) -> Error_Confirmed : [ErrCdn == 1 ]
  Error_Confirmed -> (junction 25)
  data: Err_B_Detd output; ErrCdn input; DetnDly input

== stateflow chart sub1/EmInvCtrl/Chart ==
  state Init
    entry:
    VMC_EmInvMod_Zs_Reqd = 0;
  note: Req. 44, 45
  note: 39. The function shall request that the inverters enter operational mode in PM3 after the Inverters report that they are in PreOp mode
  state OpMode_Req
    entry:
    VMC_EmInvMod_Zs_Reqd = 1;
  (default) -> Init
  OpMode_Req -> Init : [VMC_PwrMod_Zs ~= 3]
      | % Power mode not equal to 3
  Init -> OpMode_Req : [EX_RiEmInvMod_Zs == 127 ... % Inv in Pre-Op mode
      | && EX_LeEmInvMod_Zs == 127 ... % Inv in Pre-Op mode
      | && VMC_PwrMod_Zs == 3] % Power mode equal to 3
  data: EX_LeEmInvMod_Zs input; EX_RiEmInvMod_Zs input; VMC_PwrMod_Zs input; VMC_EmInvMod_Zs_Reqd output

== stateflow chart sub1/HiVoltBatCtrl/Chart ==
  state LOW
    entry:
    VMC_HiVoltBatt_B_Enad = 0;
  note: 40. The function shall delay the HV battery enable by a calibratable duration after the VCU goes live.
  state HIGH
    entry:
    VMC_HiVoltBatt_B_Enad = 1;
  (default) -> LOW
  HIGH -> LOW : [VMC_EcuShtdn_B_Reqd]
  LOW -> HIGH : [after (HiVoltBatEnaDly_T_Pt, sec)] % After Cal delay time
  data: HiVoltBatEnaDly_T_Pt input; VMC_EcuShtdn_B_Reqd input; VMC_HiVoltBatt_B_Enad output

== stateflow chart sub1/HiVoltBatCtrl/HiVoltBatModeReq ==
  state Disconnect
    entry:
    HiVoltBatMod_Zs_Reqd = 0;
  note: 32. The function shall request the battery to disconnect when:
      | 1. The key switch goes low
      | 2. CTM shutdown inhibit is low
  note: 31. The function shall request the battery to connect for driving in PM1 after The battery reports "Disconnected, awaiting HV request"
  note: 43. The function shall only request for the HV battery to connect for driving when the inverters report that they have disabled active discharge
  state ConnectForDriving
    entry:
    HiVoltBatMod_Zs_Reqd = 16
  (default) -> Disconnect
  ConnectForDriving -> Disconnect : [
      | ~EX_KeySwt_B_Enad ... % KeySwt LOW
      | && ~CTM_EcuShtdn_B_Inhtd
      | ]
  Disconnect -> ConnectForDriving : [
      | VMC_PwrMod_Zs == 1 ...
      | && EX_HiVoltBatSts_Zs == 3 ...
      | && EX_RiEmInvActvDcha_B_Enad ==0 ...
      | && EX_LeEmInvActvDcha_B_Enad ==0
      | ]
  data: EX_KeySwt_B_Enad input; VMC_PwrMod_Zs input; HiVoltBatMod_Zs_Reqd output; CTM_EcuShtdn_B_Inhtd input; EX_HiVoltBatSts_Zs input; EX_RiEmInvActvDcha_B_Enad input; EX_LeEmInvActvDcha_B_Enad input

== stateflow chart sub1/HiVoltBatCtrl/Time/Hour/CountTo24 ==
  state initialise
    entry:
    Out = 0;
  state AddOne
    entry:
    Out = Out + In;
  (default) -> initialise
  (junction 2) -> initialise
  (junction 4) -> (junction 2) : [Out >= 24]
  initialise -> AddOne : [In == 1]
  AddOne -> AddOne [order 2]
  AddOne -> (junction 4) [order 1]
  data: In input; Out output

== stateflow chart sub1/PwrMod ==
  note: 2. When the ECU is turned on, it shall enter either PM1 or PM4 based on: Active system HW mode (Charge or Drive)
  state Power_Modes
    state PM_1
      % Legacy 24v system connected
      % (KL15 connected and battery initialised)
      entry:
      VMC_PwrMod_Zs = 1;
    note: 27. The PM1 to PM2 transition shall occur when:
        | 1. The accessory button is pressed
        | 2. HV battery is connected for driving
    note: 18. The function shall ensure that all HV loads are switched off before transitioning to PM4
    note: 29. The function shall transition to PM1 from PM2 or PM3 when the accessory button goes low and vehicle is stationary
    state PM_2
      % Preparing torque availability.
      % (KL15 connected and checks commence)
      entry:
      VMC_PwrMod_Zs = 2;
    state PM_4
      % Charging mode
      entry:
      VMC_PwrMod_Zs = 4;
    state Turn_off_Hv_Loads
      entry:
      VMC_HiVoltLoaOff_B_Reqd = 1;
      %Request all HV loads off
    note: Req. 8
    note: 3. When the charger is inserted, the system shall transition to PM4 when:
        | a) Vehicle is stationary
        | b) System is in PM 0,1, or 2
    note: 8. The function shall transition from PM2 to PM3 when the following conditions are true:
        | a) HV battery connected for driving
        | b) Air system precharge complete and within range
        | c) A minimum duration has passed
        | d) Gear in Neutral
        | e) Brake is depressed
        | f) No drive inhibit flags set by FR
        | g) The start button is pressed
    note: 4. When the charger is removed and ignition is ON, then the system shall remain in PM4 .
    note: Req. 8
    note: 5. When the system is stuck in PM4 after the charger has been removed with ignition ON, a reset of the ignition will be required to leave PM4.
    state PM_3
      % Torque available and power meter displayed
      % (Checks completed successfully)
      entry:
      VMC_PwrMod_Zs = 3;
    (junction 110) -> PM_1
    PM_1 -> (junction 123) [order 2]
    (junction 108) -> (junction 110) : [
        | CSE_IgKeyPosn_Zs == 0 ... % Accesorry button LOW
        | && CSE_VehStaty_B ... %Vehicle stationary
        |  ]
    (junction 123) -> (junction 125)
    PM_1 -> PM_2 [order 1] : [
        | CSE_IgKeyPosn_Zs == 1 ... % Accessory button High
        | && EX_HiVoltBatSts_Zs == 21 % Battery connected for driving
        | ]
    PM_2 -> (junction 108) [order 3]
    PM_2 -> (junction 125) [order 1]
    (junction 125) -> Turn_off_Hv_Loads : [EX_Chrgr_B_Cnnct]
    (junction 115) -> (junction 108)
    Turn_off_Hv_Loads -> PM_4 : [
        | EPC_HiVoltLoaOff_B...
        | && CSE_VehStaty_B
        | ]
    PM_2 -> (junction 88) [order 2] : [
        | after (SteerPDly_T_Pt, sec)
        | % Minimum duration
        | ]
    (junction 88) -> PM_3 : [
        | EX_HiVoltBatSts_Zs == 21 ... % HV battery connected for driving
        | && SPC_IniPChrgSts_B ... % Initial pressurisation complete
        | && EX_PrimResvr_Pbar > SplyResvr_Pbar_Min_Pt ... % Prim Tank pressure above min
        | && EX_SecryResvr_Pbar > SplyResvr_Pbar_Min_Pt ... % Sec Tank pressure above min
        | && VMC_EltGearPosn_Zs == 0 ... % Gear in Neutral
        | && DPD_BrkPedl_B_Depr ... %Brake depressed
        | && ~FR_Drv_B_Inhtd ... No drive inhibit flags set
        | && CSE_IgKeyPosn_Zs == 3 ... % Crank button high
        | ]
    PM_3 -> (junction 115)
  (default) -> (junction 74)
  (junction 74) -> (junction 76) [order 1]
  (junction 74) -> PM_1 [order 2] : % Drive mode
  (junction 76) -> Turn_off_Hv_Loads : [CSE_SysHwMod_Zs ==1 ]
      | % Charge mode
  data: VMC_PwrMod_Zs output; EX_Chrgr_B_Cnnct input; CSE_SysHwMod_Zs input; SPC_IniPChrgSts_B input; SteerPDly_T_Pt input; EX_HiVoltBatSts_Zs input; CSE_IgKeyPosn_Zs input; VMC_HiVoltLoaOff_B_Reqd output; VMC_EltGearPosn_Zs input; SplyResvr_Pbar_Min_Pt input; FR_Drv_B_Inhtd input; EX_SecryResvr_Pbar input; EX_PrimResvr_Pbar input; EPC_HiVoltLoaOff_B input; DPD_BrkPedl_B_Depr input; CSE_VehStaty_B input
